simulink model "week1problem4"  (R2020b)
settings: Solver=VariableStepAuto  StartTime=0.0  StopTime=10.0  RelTol=1e-3
libraries: dspsrcs4 x1
settings Model: Creator=Puru Gawande  LastModifiedBy=Puru Gawande

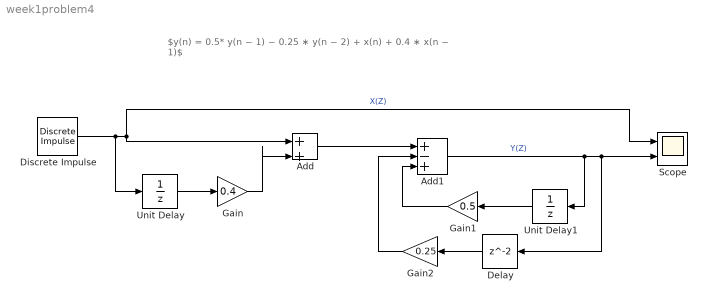
== system week1problem4 ==
  note: $y(n) = 0.5* y(n − 1) − 0.25 ∗ y(n − 2) + x(n) + 0.4 ∗ x(n − 1)$
  Add : Sum  Inputs=++|
  Add1 : Sum  Inputs=+-+
  Delay : Delay
  Discrete Impulse : dspsrcs4/Discrete  Impulse  Delay=5  SampleTime=0.5  FrameSample=1  OutputFrames=off  dataType=double  isSigned=on  wordLen=16  udDataType=sfix(16)  fracBitsMode=Best precision  numFracBits=15  OutDataTypeStr=double  LastOutDataTypeStr=double
  Gain : Gain  Gain=0.4
  Gain1 : Gain  Gain=0.5
  Gain2 : Gain  Gain=0.25
  Scope : Scope  NumInputPorts=2
  Unit Delay : UnitDelay  SampleTime=-1  HasFrameUpgradeWarning=on
  Unit Delay1 : UnitDelay  SampleTime=-1  HasFrameUpgradeWarning=on
  wires:
  Discrete Impulse/1 -> Unit Delay/1, Scope/1, Add/1  "X(Z)"
  Unit Delay/1 -> Gain/1
  Gain/1 -> Add/2
  Add/1 -> Add1/1
  Add1/1 -> Unit Delay1/1, Delay/1, Scope/2  "Y(Z)"
  Unit Delay1/1 -> Gain1/1
  Gain1/1 -> Add1/3
  Delay/1 -> Gain2/1
  Gain2/1 -> Add1/2
